simulink model "I_Regler"  (Simulink 8.7)
settings: Solver=VariableStepAuto  StartTime=0.0  StopTime=10.0  RelTol=1e-3
values from neighbouring files (symbols this model uses):
  K = V*Km/(s1*s2*L*J)    [omega_s_to_kp.m]
  Ki = 1/tau    [time_to_sum_form.m]
  tau1 = -1/s1    [omega_s_to_kp.m]
undefined symbols (not defined in the file or in its folder): tau2
settings Model: Creator=Andreas  LastModifiedBy=Andreas
settings DataIOCC: LimitDataPoints=off  SaveFormat=Dataset
settings DebuggingCC: UnderspecifiedInitializationDetection=Simplified  MergeDetectMultiDrivingBlocksExec=error
settings HardwareCC: ProdBitPerPointer=64  ProdLargestAtomicFloat=Float  ProdIntDivRoundTo=Zero  ProdEndianess=LittleEndian  ProdWordSize=64  ProdHWDeviceType=Intel->x86-64 (Windows64)
settings ModelReferenceCC: PropagateSignalLabelsOutOfModel=on
settings ConfigComp: CovModelRefEnable=off

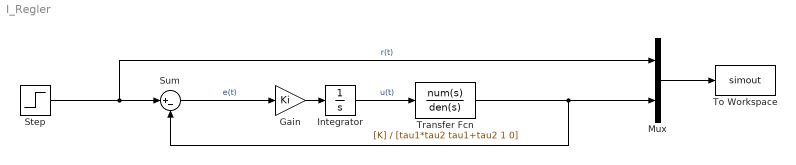
== system I_Regler ==
  Gain : Gain  Gain=Ki
  Integrator : Integrator
  Mux : Mux  Inputs=2
  Step : Step  SampleTime=0
  Sum : Sum  Inputs=|+-
  To Workspace : ToWorkspace  VariableName=simout  SaveFormat=Structure With Time  SampleTime=-1
  Transfer Fcn : TransferFcn  Numerator=[K]  Denominator=[tau1*tau2 tau1+tau2 1 0]
  wires:
  Step/1 -> Mux/1, Sum/1  "r(t)"
  Sum/1 -> Gain/1  "e(t)"
  Gain/1 -> Integrator/1
  Integrator/1 -> Transfer Fcn/1  "u(t)"
  Transfer Fcn/1 -> Sum/2, Mux/2
  Mux/1 -> To Workspace/1
